simulink model "DAQ_v7_IMU_no_Boom_improved_differentiation"  (Simulink 7.8)
settings: Solver=ode3  StartTime=0.0  StopTime=inf  FixedStep=0.001  RelTol=1e-3
InitFcn:
  | DAQParams
model workspace: external: MATLAB File (data not in the file)
undefined symbols (not defined in the file or in its folder): A_dirty_deriv, A_dirty_deriv_IMU, B_dirty_deriv, B_dirty_deriv_IMU, C_dirty_deriv, C_dirty_deriv_IMU, CalParams, D_dirty_deriv, D_dirty_deriv_IMU, Dt_dirty_deriv, Dt_dirty_deriv_IMU, IMU_Alignment_Params, MotorParams, x0_dirty_deriv, x0_dirty_deriv_IMU
libraries: xpcethercatlib x169, dspswit3 x1
(part 3 of 3)

== matlab function DAQ/calibrate_and_convert_to_rad ==
  data: params input double; u input double; y output double
function y = calibrate_and_convert_to_rad(params,u)
%#eml
%This function calibrates the encoder values and converts to radians. The
%calibration is based on the measurements and values given by OSU, as
%listed at http://code.google.com/p/atrias/source/browse/robot_definitions/
% -Our left leg is a type 3 leg, and our right leg is a type 4 leg
% -In OSU terminology, A=shin and B=thigh
% -In UMich terminology, 1=shin and 2=thigh
% -In OSU terminology, Leg=shin/thigh encoder and Trans=motor encoder (i.e.
%         our q_gr1R, etc.)
% -The inputs and outputs are expressed in UMich terminology, but the
% calibration params are expressed in OSU terminology

y = zeros(15,1); %I put these in the desired order, slightly different from the input order


%The inputs, which are encoder values in ticks 
leg_1L_encoder = u(1);
motor_1L_encoder = u(2);
leg_2L_encoder = u(3);
motor_2L_encoder = u(4);
leg_1R_encoder = u(5);
motor_1R_encoder = u(6);
leg_2R_encoder = u(7);
motor_2R_encoder = u(8);
hip_abs_3R_encoder = u(9);
hip_inc_3R_encoder = u(10);
hip_abs_3L_encoder = u(11);
hip_inc_3L_encoder = u(12);
IMU_Z_angle_rad = u(13);
IMU_Y_angle_rad = u(14); 
IMU_X_angle_rad = u(15);

%The calibration parameters, given in the files at http://code.google.com/p/atrias/source/browse/robot_definitions/
%From robot_invariant_defs.h
LEG_A_CALIB_LOC = params(1); %Calibration angle in OSU convention radians, based on Solidworks; Same for Leg and Motor/Trans 
LEG_B_CALIB_LOC = params(2);  %Calibration angle in OSU convention radians, based on Solidworks; Same for Leg and Motor/Trans
PITCH_ENCODER_RAD_PER_TICK = params(3); %Ticks to rad constant
HIP_INC_ENCODER_RAD_PER_TICK = params(4);  %Ticks to rad constant
HIP_ABS_ENCODER_RAD_PER_TICK = params(5); %Ticks to rad constant
%From biped2_variant_defs.h
LEFT_HIP_CALIB_VAL = params(6);   %Calibration encoder value in ticks (OSU convention)
RIGHT_HIP_CALIB_VAL = params(7);  %Calibration encoder value in ticks (OSU convention)
LEFT_HIP_CALIB_POS = params(8);  %Calibration angle in radians (OSU convention)
RIGHT_HIP_CALIB_POS = params(9); %Calibration angle in radians (OSU convention)
BOOM_PITCH_VERTICAL_VALUE = params(10); %The pitch encoder's reading (in ticks) when the robot is vertical
BOOM_X_METERS_PER_TICK = params(11); %The meters of boom motion per encoder tick. This is calculated from the boom's length, the number of encoder ticks per encoder revolution, and the gear ratio between the boom and the encoder.
%From leg3_definitions.h (corresponds to our left leg)
%(Note that A=shin and B=thigh for OSU convention)
LEG3_LEG_A_CALIB_VAL = params(12); %Calibration encoder value in ticks
LEG3_LEG_B_CALIB_VAL = params(13); %Calibration encoder value in ticks
LEG3_LEG_A_RAD_PER_CNT = params(14); %Ticks to rad constant
LEG3_LEG_B_RAD_PER_CNT = params(15); %Ticks to rad constant
LEG3_TRAN_A_CALIB_VAL = params(16); %Calibration encoder value in ticks
LEG3_TRAN_B_CALIB_VAL = params(17); %Calibration encoder value in ticks
LEG3_TRAN_A_RAD_PER_CNT = params(18); %Ticks to rad constant
LEG3_TRAN_B_RAD_PER_CNT = params(19); %Ticks to rad constant
%From leg4_definitions.h (corresponds to our right leg)
%(Note that A=shin and B=thigh for OSU convention)
LEG4_LEG_A_CALIB_VAL = params(20); %Calibration encoder value in ticks
LEG4_LEG_B_CALIB_VAL = params(21); %Calibration encoder value in ticks
LEG4_LEG_A_RAD_PER_CNT = params(22); %Ticks to rad constant
LEG4_LEG_B_RAD_PER_CNT = params(23); %Ticks to rad constant
LEG4_TRAN_A_CALIB_VAL = params(24); %Calibration encoder value in ticks
LEG4_TRAN_B_CALIB_VAL = params(25); %Calibration encoder value in ticks
LEG4_TRAN_A_RAD_PER_CNT = params(26); %Ticks to rad constant
LEG4_TRAN_B_RAD_PER_CNT = params(27); %Ticks to rad constant

%%%%%%This next part is a hack, to be used until we get the absolute hip
%%%%%%encoders working
HIP_INC_CALIB_VAL = params(28); %This is UMich calibration value in radians; assumes that the robot starts out with legs at the "folded in" position
LEFT_HIP_INC_CALIB_CNT = params(29); %This is UMich calibration value in ticks (for UMich left hip incremental encoder)
RIGHT_HIP_INC_CALIB_CNT = params(30); %This is UMich calibration value in ticks (for UMich right hip incremental encoder)
HIP_INC_MAX_ENCODER_TICKS = params(31); %Max value of the incremental hip encoder

%Calibrate and convert leg_1R encoder
leg_1R_cal_set_pt_rad = LEG_A_CALIB_LOC;
leg_1R_cal_set_pt_ticks = LEG4_LEG_A_CALIB_VAL;
leg_1R_ticks_to_rad_const = LEG4_LEG_A_RAD_PER_CNT;
y(1) = calibrate_abs_encoder(leg_1R_cal_set_pt_rad,leg_1R_cal_set_pt_ticks,leg_1R_ticks_to_rad_const,leg_1R_encoder);

%Calibrate and convert motor_1R encoder
motor_1R_cal_set_pt_rad = LEG_A_CALIB_LOC;
motor_1R_cal_set_pt_ticks = LEG4_TRAN_A_CALIB_VAL;
motor_1R_ticks_to_rad_const = LEG4_TRAN_A_RAD_PER_CNT;
y(2) = calibrate_abs_encoder(motor_1R_cal_set_pt_rad,motor_1R_cal_set_pt_ticks,motor_1R_ticks_to_rad_const,motor_1R_encoder);

%Calibrate and convert leg_2R encoder
leg_2R_cal_set_pt_rad = LEG_B_CALIB_LOC;
leg_2R_cal_set_pt_ticks = LEG4_LEG_B_CALIB_VAL;
leg_2R_ticks_to_rad_const = LEG4_LEG_B_RAD_PER_CNT;
y(3) = calibrate_abs_encoder(leg_2R_cal_set_pt_rad,leg_2R_cal_set_pt_ticks,leg_2R_ticks_to_rad_const,leg_2R_encoder);

%Calibrate and convert motor_2R encoder
motor_2R_cal_set_pt_rad = LEG_B_CALIB_LOC;
motor_2R_cal_set_pt_ticks = LEG4_TRAN_B_CALIB_VAL;
motor_2R_ticks_to_rad_const = LEG4_TRAN_B_RAD_PER_CNT;
y(4) = calibrate_abs_encoder(motor_2R_cal_set_pt_rad,motor_2R_cal_set_pt_ticks,motor_2R_ticks_to_rad_const,motor_2R_encoder);

%Calibrate and convert leg_1L encoder
leg_1L_cal_set_pt_rad = LEG_A_CALIB_LOC;
leg_1L_cal_set_pt_ticks = LEG3_LEG_A_CALIB_VAL;
leg_1L_ticks_to_rad_const = LEG3_LEG_A_RAD_PER_CNT;
y(5) = calibrate_abs_encoder(leg_1L_cal_set_pt_rad,leg_1L_cal_set_pt_ticks,leg_1L_ticks_to_rad_const,leg_1L_encoder);

%Calibrate and convert motor_1L encoder
motor_1L_cal_set_pt_rad = LEG_A_CALIB_LOC;
motor_1L_cal_set_pt_ticks = LEG3_TRAN_A_CALIB_VAL;
motor_1L_ticks_to_rad_const = LEG3_TRAN_A_RAD_PER_CNT;
y(6) = calibrate_abs_encoder(motor_1L_cal_set_pt_rad,motor_1L_cal_set_pt_ticks,motor_1L_ticks_to_rad_const,motor_1L_encoder);

%Calibrate and convert leg_2L encoder
leg_2L_cal_set_pt_rad = LEG_B_CALIB_LOC;
leg_2L_cal_set_pt_ticks = LEG3_LEG_B_CALIB_VAL;
leg_2L_ticks_to_rad_const = LEG3_LEG_B_RAD_PER_CNT;
y(7) = calibrate_abs_encoder(leg_2L_cal_set_pt_rad,leg_2L_cal_set_pt_ticks,leg_2L_ticks_to_rad_const,leg_2L_encoder);

%Calibrate and convert motor_2L encoder
motor_2L_cal_set_pt_rad = LEG_B_CALIB_LOC;
motor_2L_cal_set_pt_ticks = LEG3_TRAN_B_CALIB_VAL;
motor_2L_ticks_to_rad_const = LEG3_TRAN_B_RAD_PER_CNT;
y(8) = calibrate_abs_encoder(motor_2L_cal_set_pt_rad,motor_2L_cal_set_pt_ticks,motor_2L_ticks_to_rad_const,motor_2L_encoder);

%Calibrate and convert hip_abs_3R_encoder
hip_abs_3R_cal_set_pt_rad = LEFT_HIP_CALIB_POS; %Michigan right is OSU left
hip_abs_3R_cal_set_pt_ticks = LEFT_HIP_CALIB_VAL; %Michigan right is OSU left
hip_abs_3R_ticks_to_rad_const = HIP_ABS_ENCODER_RAD_PER_TICK;
y(9) = calibrate_abs_encoder(hip_abs_3R_cal_set_pt_rad,hip_abs_3R_cal_set_pt_ticks,hip_abs_3R_ticks_to_rad_const,hip_abs_3R_encoder);

%Calibrate and convert hip_inc_3R_encoder (In essence, we're just setting
%the folded in hip position to correspond to HIP_INC_CALIB_VAL)
hip_inc_3R_cal_set_pt_rad = HIP_INC_CALIB_VAL; 
hip_inc_3R_cal_set_pt_ticks = RIGHT_HIP_INC_CALIB_CNT;
hip_inc_3R_ticks_to_rad_const = HIP_INC_ENCODER_RAD_PER_TICK;
hip_inc_3R_max_encoder_ticks = HIP_INC_MAX_ENCODER_TICKS;
y(10) = convert_inc_encoder_with_rollover(hip_inc_3R_max_encoder_ticks,hip_inc_3R_cal_set_pt_rad,hip_inc_3R_cal_set_pt_ticks,hip_inc_3R_ticks_to_rad_const,hip_inc_3R_encoder);

%Calibrate and convert hip_abs_3L_encoder
hip_abs_3L_cal_set_pt_rad = RIGHT_HIP_CALIB_POS; %Michigan left is OSU right
hip_abs_3L_cal_set_pt_ticks = RIGHT_HIP_CALIB_VAL; %Michigan left is OSU right
hip_abs_3L_ticks_to_rad_const = HIP_ABS_ENCODER_RAD_PER_TICK;
y(11) = calibrate_abs_encoder(hip_abs_3L_cal_set_pt_rad,hip_abs_3L_cal_set_pt_ticks,hip_abs_3L_ticks_to_rad_const,hip_abs_3L_encoder);

%Calibrate and convert hip_inc_3L_encoder (In essence, we're just setting
%the folded in hip position to correspond to HIP_INC_CALIB_VAL)
hip_inc_3L_cal_set_pt_rad = HIP_INC_CALIB_VAL; 
hip_inc_3L_cal_set_pt_ticks = LEFT_HIP_INC_CALIB_CNT;
hip_inc_3L_ticks_to_rad_const = HIP_INC_ENCODER_RAD_PER_TICK;
hip_inc_3L_max_encoder_ticks = HIP_INC_MAX_ENCODER_TICKS;
y(12) = convert_inc_encoder_with_rollover(hip_inc_3L_max_encoder_ticks,hip_inc_3L_cal_set_pt_rad,hip_inc_3L_cal_set_pt_ticks,hip_inc_3L_ticks_to_rad_const,hip_inc_3L_encoder);

%Pass IMU angles directly through; calibration is taken care of at the level of the IMU block
y(13) = IMU_Z_angle_rad;
y(14) = IMU_Y_angle_rad; 
y(15) = IMU_X_angle_rad;
end

function calibrated_angle_in_rad = calibrate_abs_encoder(cal_set_pt_rad,cal_set_pt_ticks,ticks_to_rad_const,encoder_value_ticks)
   tick_difference = encoder_value_ticks-cal_set_pt_ticks;
   rad_difference = tick_difference*ticks_to_rad_const;
   calibrated_angle_in_rad = cal_set_pt_rad + rad_difference;
end

function calibrated_angle_in_rad = convert_inc_encoder_with_rollover(max_encoder_ticks,cal_set_pt_rad,cal_set_pt_ticks,ticks_to_rad_const,encoder_value_ticks)
    tick_difference_temp = encoder_value_ticks-cal_set_pt_ticks;
    %This part is a bit of a hack; the threshhold values work for our
    %application, but this is not exactly elegant. It's based on
    %understanding the range of our incremental encoder
    %If the difference in values is large enough, we assume that there are rollover issues 
    if tick_difference_temp > 50000 %When the cal value is a small number and the current encoder value is a large value near the rollover point 
        tick_difference = -mod(-tick_difference_temp,max_encoder_ticks);
    elseif tick_difference_temp < -5000 %This only happens when the cal value is a large value near the rollover point  
        tick_difference = mod(tick_difference_temp,max_encoder_ticks);
    else
        tick_difference = tick_difference_temp;
    end
    rad_difference = tick_difference*ticks_to_rad_const;
    calibrated_angle_in_rad = cal_set_pt_rad + rad_difference;
end

== matlab function DAQ/convert_mtr_torque_cmd_to_pwm ==
  data: params input double; u input double; y output double
function y = convert_to_pwm(params,u)
%#eml
%This function takes motor torque command inputs and outputs
%pwm commands (for the Medulla) in UMich convention

y = zeros(6,1);

%The inputs, which are commanded motor torques 
leg_motor_1R_torque_cmd = u(1);
leg_motor_2R_torque_cmd = u(2);
hip_motor_3R_torque_cmd = u(3);
leg_motor_1L_torque_cmd = u(4);
leg_motor_2L_torque_cmd = u(5);
hip_motor_3L_torque_cmd = u(6);

%Parameters determined experimentally at U Mich
UMich_LEFT_MOTOR_HIP_DIRECTION = params(1); %The direction for the left hip motor. (UMich convention)
UMich_RIGHT_MOTOR_HIP_DIRECTION = params(2); %The direction for the right hip motor. (UMich convention)

% The parameters, from http://code.google.com/p/atrias/source/browse/robot_definitions/
%From robot_invariant_defs.h
MTR_MAX_COUNT = params(3); %The maximum commanded amplifier value. This is the maximum value sent to the Medullas for the amplifier command.
%From biped2_variant_defs.h
MTR_MAX_TORQUE = params(4); %Maximum motor torque for scaling
MTR_HIP_MAX_TORQUE = params(5); %Maximum hip motor torque for scaling
%From leg3_definitions.h (corresponds to our left leg)
%(Note that A=shin and B=thigh for OSU convention)
LEG3_MOTOR_A_DIRECTION = params(6);
LEG3_MOTOR_B_DIRECTION = params(7);
%From leg4_definitions.h (corresponds to our right leg)
%(Note that A=shin and B=thigh for OSU convention)
LEG4_MOTOR_A_DIRECTION = params(8);
LEG4_MOTOR_B_DIRECTION = params(9);

leg_torque_to_pwm = MTR_MAX_COUNT/MTR_MAX_TORQUE;
hip_torque_to_pwm = MTR_MAX_COUNT/MTR_HIP_MAX_TORQUE;

%Convert leg_motor_1L_torque_cmd
leg_motor_1L_direction = LEG3_MOTOR_A_DIRECTION;
y(1) = motor_torque_to_pwm(leg_motor_1L_direction,leg_torque_to_pwm,leg_motor_1L_torque_cmd);

%Convert leg_motor_2L_torque_cmd
leg_motor_2L_direction = LEG3_MOTOR_B_DIRECTION;
y(2) = motor_torque_to_pwm(leg_motor_2L_direction,leg_torque_to_pwm,leg_motor_2L_torque_cmd);

%Convert leg_motor_1R_torque_cmd
leg_motor_1R_direction = LEG4_MOTOR_A_DIRECTION;
y(3) = motor_torque_to_pwm(leg_motor_1R_direction,leg_torque_to_pwm,leg_motor_1R_torque_cmd);

%Convert leg_motor_2R_torque_cmd
leg_motor_2R_direction = LEG4_MOTOR_B_DIRECTION;
y(4) = motor_torque_to_pwm(leg_motor_2R_direction,leg_torque_to_pwm,leg_motor_2R_torque_cmd);

%Convert hip_motor_3R_torque_cmd
hip_motor_3R_direction = UMich_RIGHT_MOTOR_HIP_DIRECTION; %Verified experimentally
y(5) = motor_torque_to_pwm(hip_motor_3R_direction,hip_torque_to_pwm,hip_motor_3R_torque_cmd);

%Convert hip_motor_3L_torque_cmd
hip_motor_3L_direction = UMich_LEFT_MOTOR_HIP_DIRECTION; %Verified experimentally
y(6) = motor_torque_to_pwm(hip_motor_3L_direction,hip_torque_to_pwm,hip_motor_3L_torque_cmd);

end

function motor_pwm = motor_torque_to_pwm(motor_direction,torque_to_pwm_const,motor_torque_cmd)
   motor_pwm = motor_direction*torque_to_pwm_const*motor_torque_cmd;
end
